simulink model "ansiBPF"  (R2018a)
settings: Solver=VariableStepAuto  StartTime=0.0  StopTime=0.001  RelTol=1e-3
undefined symbols (not defined in the file): fdesignblkfcn, G1, G10, G11, G12, G13, G14, G15, G16, G17, G18, G19, G2, G20, G21, G22, G23, G24, G25, G26, G3, G4, G5, G6, G7, G8, G9, gcbh, get, T
libraries: dspsrcs4 x1, dspxfrm3 x1, dspobslib x1
(part 5 of 8)

== system ansiBPF/Filter Bank /Filter 25/Bandpass Filter ==
  In : Inport
  Generated Filter Block : DiscreteFir  Tag=BlockMethodSubSystem  Coefficients=[-0.00381457351441647202 0.00633341068892222161 0.00335056419677833527 -0.018442727442746748 0.0129728943442847921 0.0119081702309962734 -0.0179320505622532177 0.00126041430991428657 -0.0118297034124350275 0.0438106024069588665 -0.00275448548765090673 -0.114954073416214858 0.130994387812402524 0.0558760887693779407 -0.23385262110053362 0.136677561279248183 0.136677561279248183 -0.23385262110053362 0.0558760887693779407 0.130994387812402524 -0.114954073416214858 -0.00275448548765090673 0.0438106024069588665 -0.0118297034124350275 0.00126041430991428657 -0.0179320505622532177 0.0119081702309962734 0.0129728943442847921 -0.018442727442746748 0.00335056419677833527 0.00633341068892222161 -0.00381457351441647202]  InputProcessing=Columns as channels (frame based)
  Out : Outport
  wires:
  In/1 -> Generated Filter Block/1
  Generated Filter Block/1 -> Out/1

== system ansiBPF/Filter Bank /Filter 26/Bandpass Filter ==
  In : Inport
  Generated Filter Block : DiscreteFir  Tag=BlockMethodSubSystem  Coefficients=[-0.0030943355205251895 0.00909935305967807771 -0.0160738281165847922 0.0189403165077401021 -0.0141093398046298335 0.00433830456128312791 0.00112563970749806589 0.00629989940724654321 -0.0250159563306298835 0.0411554128755461657 -0.0391179700810540126 0.017802342331145974 0.00306610844812084176 0.00329129629654466684 -0.0445397426369277122 0.0933261269325897092 -0.100299771613024724 0.0314673704549710415 0.098396444865320315 -0.226161269375300594 0.279325502164850636 -0.226161269375300594 0.098396444865320315 0.0314673704549710415 -0.100299771613024724 0.0933261269325897092 -0.0445397426369277122 0.00329129629654466684 0.00306610844812084176 0.017802342331145974 -0.0391179700810540126 0.0411554128755461657 -0.0250159563306298835 0.00629989940724654321 0.00112563970749806589 0.00433830456128312791 -0.0141093398046298335 0.0189403165077401021 -0.0160738281165847922 0.00909935305967807771 -0.0030943355205251895]  InputProcessing=Columns as channels (frame based)
  Out : Outport
  wires:
  In/1 -> Generated Filter Block/1
  Generated Filter Block/1 -> Out/1

== system ansiBPF/Filter Bank /Filter 3/Bandpass Filter ==
  In : Inport
  Generated Filter Block : DiscreteFir  Tag=BlockMethodSubSystem  Coefficients=[-0.00623302073745927651 -0.000147156546448560485 -0.000148497532856758593 -0.000150537315393745692 -0.000151851403328953996 -0.000153865058740236272 -0.000155131168425097683 -0.000157111777232369509 -0.000158316640811846708 -0.000160247025504315537 -0.000161364375664084118 -0.000163235311863951836 -0.000164236368263929311 -0.000166016533083678279 -0.000166870520616942955 -0.00016854077674887912 -0.000169207289079283807 -0.000170747001524051864 -0.000171185027124507388 -0.000172584370149106149 -0.00017275625285197182 -0.000174025063343233777 -0.00017390126871303239 -0.000175106048418890737 -0.000174685108078305337 -0.000175967174250019894 -0.000175298264829811104 -0.000177027270963877242 -0.000176228847867884335 -0.000179405891800066242 -0.000178711609326296197 -0.000188958916936491852 -0.000178912970163004468 -0.000176144497877943476 -0.000181042774326621478 -0.000178795394882798374 -0.000180516010236460284 -0.000179074006666288466 -0.000180011884870085565 -0.000178837262190874937 -0.000179358425150408219 -0.000178271210113030762 -0.000178510333837117235 -0.000177425543832754996 -0.000177425742050259634 -0.000176292483626708355 -0.000176078798820710809 -0.000174846880596543045 -0.000174418815969579362 -0.000173043429281363064 -0.000172393454714019301 -0.000170834603616727129 -0.000169958585447208807 -0.000168190868462014977 -0.000167118464140832384 -0.000165153755473033275 -0.000163949549043370052 -0.000161861214483874848 -0.000160695164391341772 -0.00015859694805247379 -0.000157727851105920498 -0.000155634333340207495 -0.000155286706362275939 -0.000151224975015565777 -0.000147429465809554368 -0.000147673868998559981 -0.000144268865643743178 -0.000142358755707297122 -0.000139468548609581822 -0.000137138429318845693 -0.000134246976289315777 -0.000131648936936103542 -0.000128669922581075891 -0.000125862490280859526 -0.000122764874243647885 -0.00011975991024215688 -0.000116529001257987931 -0.000113337735393405652 -0.000109947251241021554 -0.000106559616598388471 -0.000102985095899570258 -9.93862222590612398e-05 -9.56038161028881619e-05 -9.1782255404333421e-05 -8.77830589487374891e-05 -8.37550165965218865e-05 -7.95653777854079522e-05 -7.53699996865678771e-05 -7.106653172258175e-05 -6.67996780903094297e-05 -6.2453694695293051e-05 -5.81574491615910984e-05 -5.37056482301179072e-05 -4.91175872768226084e-05 -4.39066078192214978e-05 -3.7969207607889703e-05 -3.45421236021801968e-05 -2.89163561604173128e-05 -2.38083062594662666e-05 -1.85381427937428277e-05 -1.32197423265283667e-05 -7.79649339975905259e-06 -2.29764063978883666e-06 3.2807917054743235e-06 8.94182087945100663e-06 1.46719338060634048e-05 2.04953196069415892e-05 2.6370906605635691e-05 3.23487762700181035e-05 3.83827875609699096e-05 4.45261645383206924e-05 5.072931756527221e-05 5.70512748638711789e-05 6.34357749862406054e-05 6.9944394706653463e-05 7.65067986614835754e-05 8.31856413912990646e-05 8.98917214415818731e-05 9.67072598686894412e-05 0.000103488911499773808 0.000110379207435208206 0.000117208401984176543 0.000124203133643797909 0.000131165967659036702 0.000138494168293898151 0.000145823935630485065 0.000153670762824138963 0.00016017656350110116 0.000167769790846511934 0.000175539490234398894 0.000182873719231709951 0.000190631400859327121 0.000198186867010095326 0.000206006222773604393 0.000213697194266508937 0.000221590231458462827 0.000229390650317221485 0.000237362866222187534 0.000245254526858947508 0.000253299405223364536 0.000261287730021923412 0.000269415601043183656 0.00027750159686051396 0.00028572203642979985 0.000293909909236260143 0.000302225596492006871 0.000310503460882179214 0.000318894758015488499 0.000327225812552325282 0.000335660260261246848 0.000343990462156427295 0.000352426304372235562 0.000360760908854641999 0.000369247133427802725 0.000377663694644495875 0.000386332889557422109 0.000394890860432212738 0.000403646785412241393 0.000411763627392100397 0.000420289195306783618 0.000429256594053985187 0.000437553272608428158 0.000446285193765224067 ...(+30083 chars)]  InputProcessing=Columns as channels (frame based)
  Out : Outport
  wires:
  In/1 -> Generated Filter Block/1
  Generated Filter Block/1 -> Out/1
